simulink model "QuadSumulink"  (R2015a)
settings: Solver=ode45  StartTime=0.0  StopTime=10.0  RelTol=1e-3
values from neighbouring files (symbols this model uses):
  d = 1.14 * 10^(-7)    (= 1.14e-07)    [SimulinkDataQuad.m]    (also in angularquadmodel.m)
  g = 9.81    [SimulinkDataQuad.m]    (also in calc.m; quadmodel.m)
  Ix = 4.856 * 10^(-3)    (= 0.004856)    [SimulinkDataQuad.m]
  Iy = iX    [SimulinkDataQuad.m]
  Iz = 8.801 * 10^(-3)    (= 0.008801)    [SimulinkDataQuad.m]
  jP = 0    [SimulinkDataQuad.m]    (also in angularquadmodel.m)
  k = 2.98 * 10^(-6)    (= 2.98e-06)    [SimulinkDataQuad.m]    (also in angularquadmodel.m; quadmodel.m)
  l = 0.225    [SimulinkDataQuad.m]    (also in angularquadmodel.m)
  m = 0.468    [SimulinkDataQuad.m]    (also in calc.m; quadmodel.m)
settings Model: Creator=Subhechha  LastModifiedBy=Subhechha

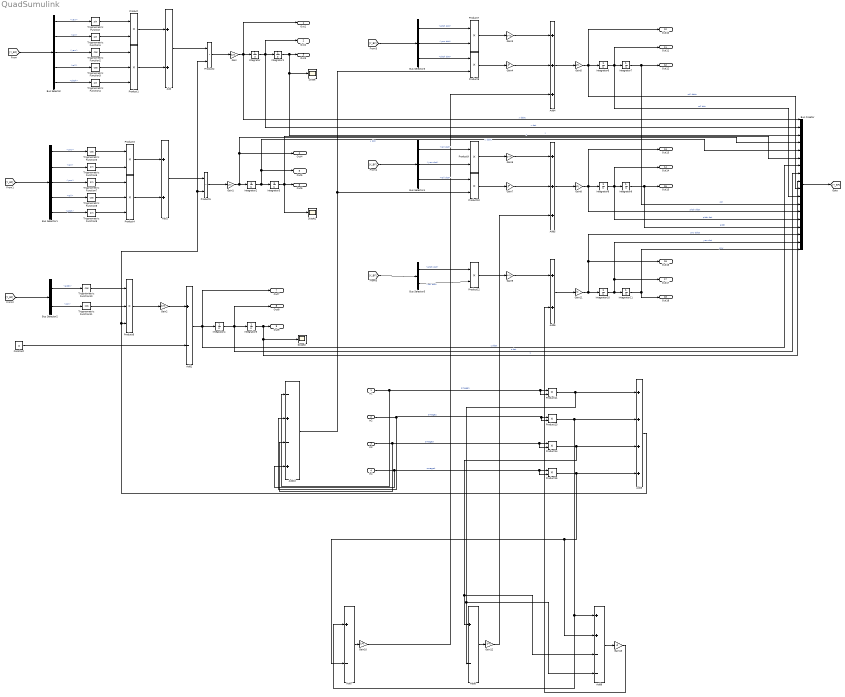
== system QuadSumulink ==
  In1 : Inport
  In2 : Inport  Port=2
  In3 : Inport  Port=3
  In4 : Inport  Port=4
  Add : Sum
  Add1 : Sum
  Add10 : Sum  Inputs=-+-+
  Add2 : Sum  Inputs=+-
  Add3 : Sum  Inputs=++++
  Add4 : Sum  Inputs=+++
  Add5 : Sum  Inputs=+++
  Add6 : Sum
  Add7 : Sum  Inputs=+-
  Add8 : Sum  Inputs=+-
  Add9 : Sum  Inputs=++--
  Bus Creator : BusCreator  Inputs=18
  Bus Selector : BusSelector  OutputSignals=yaw,roll,yaw,roll,pitch
  Bus Selector1 : BusSelector  OutputSignals=yaw,roll,yaw,roll,pitch
  Bus Selector2 : BusSelector  OutputSignals=pitch,roll
  Bus Selector3 : BusSelector  OutputSignals=pitch dot,yaw dot,pitch dot
  Bus Selector4 : BusSelector  OutputSignals=roll dot,yaw dot,roll dot
  Bus Selector5 : BusSelector  OutputSignals=pitch dot,roll dot
  Constant : Constant  Value=g
  Gain : Gain  Gain=k/m
  Gain1 : Gain  Gain=k/m
  Gain10 : Gain  Gain=k*l
  Gain11 : Gain  Gain=Iz
  Gain12 : Gain  Gain=k*l
  Gain13 : Gain  Gain=d
  Gain2 : Gain  Gain=k/m
  Gain3 : Gain  Gain=Iy-Iz
  Gain4 : Gain  Gain=jP
  Gain5 : Gain  Gain=1/Ix
  Gain6 : Gain  Gain=Iz-Ix
  Gain7 : Gain  Gain=jP
  Gain8 : Gain  Gain=1/Iy
  Gain9 : Gain  Gain=Ix-Iy
  Integrator{,1..11} (12 alike) : Integrator
  Product{,2..3,5,7..15} (13 alike) : Product
  Product1 : Product  Inputs=3
  Product4 : Product  Inputs=3
  Product6 : Product  Inputs=3
  Scope : Scope
  Scope1 : Scope
  Scope2 : Scope
      settings: SaveName=ScopeData2
  Trigonometric Function{,1,4,6..7,9} (6 alike) : Trigonometry
  Trigonometric Function{2..3,5,8,10..11} (6 alike) : Trigonometry  Operator=cos
  Out1 : Outport
  Out2 : Outport  Port=2
  Out3 : Outport  Port=3
  Out4 : Outport  Port=4
  Out5 : Outport  Port=5
  Out6 : Outport  Port=6
  Out7 : Outport  Port=7
  Out8 : Outport  Port=8
  Out9 : Outport  Port=9
  Out10 : Outport  Port=10
  Out11 : Outport  Port=11
  Out12 : Outport  Port=12
  Out13 : Outport  Port=13
  Out14 : Outport  Port=14
  Out15 : Outport  Port=15
  Out16 : Outport  Port=16
  Out17 : Outport  Port=17
  Out18 : Outport  Port=18
  wires:
  Trigonometric Function1/1 -> Product/2
  Trigonometric Function/1 -> Product/1
  Trigonometric Function2/1 -> Product1/1
  Trigonometric Function3/1 -> Product1/2
  Trigonometric Function4/1 -> Product1/3
  Product1/1 -> Add/2
  Product/1 -> Add/1
  Add/1 -> Product2/1
  Product2/1 -> Gain/1
  Gain/1 -> Bus Creator/1, Out1/1, Integrator/1  "x ddot"
  Integrator/1 -> Bus Creator/2, Out2/1, Integrator1/1  "x dot"
  Integrator1/1 -> Scope/1, Bus Creator/3, Out3/1  "x"
  [Y_BF] -> Bus Selector/1
  Trigonometric Function6/1 -> Product3/2
  Trigonometric Function5/1 -> Product3/1
  Trigonometric Function7/1 -> Product4/1
  Trigonometric Function8/1 -> Product4/2
  Trigonometric Function9/1 -> Product4/3
  Product4/1 -> Add1/2
  Product3/1 -> Add1/1
  Add1/1 -> Product5/1
  Product5/1 -> Gain1/1
  Gain1/1 -> Bus Creator/4, Out4/1, Integrator2/1  "y ddot"
  Integrator2/1 -> Bus Creator/5, Out5/1, Integrator3/1  "y dot"
  Integrator3/1 -> Scope1/1, Bus Creator/6, Out6/1  "y"
  [Y_BF] -> Bus Selector1/1
  Trigonometric Function10/1 -> Product6/1
  Trigonometric Function11/1 -> Product6/2
  Product6/1 -> Gain2/1
  Constant/1 -> Add2/2
  Gain2/1 -> Add2/1
  Add2/1 -> Bus Creator/7, Integrator4/1, Out7/1  "z ddot"
  Integrator4/1 -> Bus Creator/8, Integrator5/1, Out8/1  "z dot"
  Integrator5/1 -> Scope2/1, Bus Creator/9, Out9/1  "z"
  [Y_BF] -> Bus Selector2/1
  [Y_BF] -> Bus Selector3/1
  Add4/1 -> Gain5/1
  Gain5/1 -> Bus Creator/10, Integrator6/1, Out10/1  "roll ddot"
  Integrator6/1 -> Bus Creator/11, Integrator7/1, Out11/1  "roll dot"
  Integrator7/1 -> Bus Creator/12, Out12/1  "roll"
  Gain3/1 -> Add4/1
  Gain4/1 -> Add4/2
  Product8/1 -> Gain4/1
  Product7/1 -> Gain3/1
  [Y_BF] -> Bus Selector4/1
  Add5/1 -> Gain8/1
  Gain8/1 -> Out13/1, Integrator8/1, Bus Creator/13  "pitch ddot"
  Integrator8/1 -> Out14/1, Integrator9/1, Bus Creator/14  "pitch dot"
  Integrator9/1 -> Out15/1, Bus Creator/15  "pitch"
  Gain6/1 -> Add5/1
  Gain7/1 -> Add5/2
  Product10/1 -> Gain7/1
  Product9/1 -> Gain6/1
  [Y_BF] -> Bus Selector5/1
  Add6/1 -> Gain11/1
  Gain11/1 -> Integrator10/1, Bus Creator/16, Out16/1  "yaw ddot"
  Integrator10/1 -> Integrator11/1, Bus Creator/17, Out17/1  "yaw dot"
  Integrator11/1 -> Out18/1, Bus Creator/18  "yaw"
  Gain9/1 -> Add6/1
  Product12/1 -> Gain9/1
  Bus Creator/1 -> [Y_BF]
  Bus Selector/1 -> Trigonometric Function/1  "<yaw>"
  Bus Selector/2 -> Trigonometric Function1/1  "<roll>"
  Bus Selector/3 -> Trigonometric Function2/1  "<yaw>"
  Bus Selector/4 -> Trigonometric Function3/1  "<roll>"
  Bus Selector/5 -> Trigonometric Function4/1  "<pitch>"
  Bus Selector1/1 -> Trigonometric Function5/1  "<yaw>"
  Bus Selector1/2 -> Trigonometric Function6/1  "<roll>"
  Bus Selector1/3 -> Trigonometric Function7/1  "<yaw>"
  Bus Selector1/4 -> Trigonometric Function8/1  "<roll>"
  Bus Selector1/5 -> Trigonometric Function9/1  "<pitch>"
  Bus Selector2/1 -> Trigonometric Function10/1  "<pitch>"
  Bus Selector2/2 -> Trigonometric Function11/1  "<roll>"
  Bus Selector3/1 -> Product7/1  "<pitch dot>"
  Bus Selector3/2 -> Product7/2  "<yaw dot>"
  Bus Selector3/3 -> Product8/1  "<pitch dot>"
  Bus Selector4/1 -> Product9/1  "<roll dot>"
  Bus Selector4/2 -> Product9/2  "<yaw dot>"
  Bus Selector4/3 -> Product10/1  "<roll dot>"
  Bus Selector5/1 -> Product12/1  "<pitch dot>"
  Bus Selector5/2 -> Product12/2  "<roll dot>"
  In4/1 -> Add10/4, Product15/2, Product15/1  "omega4"
  In3/1 -> Add10/3, Product14/2, Product14/1  "omega3"
  In2/1 -> Product13/2, Product13/1, Add10/2  "omega2"
  In1/1 -> Add10/1, Product11/2, Product11/1  "omega1"
  Product11/1 -> Add9/4, Add8/2, Add3/1
  Product13/1 -> Add7/1, Add9/1, Add3/2
  Product15/1 -> Add9/2, Add7/2, Add3/4
  Product14/1 -> Add9/3, Add8/1, Add3/3
  Add3/1 -> Product2/2, Product5/2, Product6/3
  Add7/1 -> Gain10/1
  Gain10/1 -> Add4/3
  Add8/1 -> Gain12/1
  Gain12/1 -> Add5/3
  Add9/1 -> Gain13/1
  Gain13/1 -> Add6/2
  Add10/1 -> Product10/2, Product8/2
